simulink model "edma_single_block_transfer_profiling_s32k14x"  (Simulink 9.0)
settings: Solver=FixedStepDiscrete  StartTime=0.0  StopTime=10.0  FixedStep=2  RelTol=1e-3  EnableMultiTasking=on
model workspace (MAT data in the model file):
  dest = 1234
  sig_src = Simulink.Signal
  sig_src.DataType = 'uint32'
  sig_src.Dimensions = 1025
  sig_src.DimensionsMode = 'auto'
  sig_src.Complexity = 'auto'
  sig_src.SampleTime = -1
  sig_src.SamplingMode = 'auto'
InitFcn:
  | mbd_s32k_consistency_checks(bdroot(gcs));
undefined symbols (not defined in the file): LQFP
libraries: mbd_s32k1xx_ec_toolbox x8, simulink x1
Description:
  | Comparison betwen data transfer using eDMA and normal cpu copy.
  | 
  | Transfer sizes used are as follows:
  | 4, 8, 16, 32, 64, 128, 256, 512, 768, 1024 uint32s (multiply by 4 to get number of bytes)
  | 
  | Transfer size is changed at every step, iterating circulary over this list.
  | 
  | Verification:
  | Open freeMaster project (has the same name as the model) and observe differences betwen the 2 types of transfer.
settings Model: Creator=NXP MBDT Team  LastModifiedBy=nxf35172
settings DataIOCC: ExternalInput=off  InitialState=off  LimitDataPoints=on  SaveFormat=Dataset  SaveOutput=off  SignalLogging=off  SaveTime=off
settings OptimizationCC: DefaultParameterBehavior=Inlined  PassReuseOutputArgsAs=Individual arguments  LifeSpan=auto
settings DebuggingCC: UnderspecifiedInitializationDetection=Simplified  MergeDetectMultiDrivingBlocksExec=error  InheritedTsInSrcMsg=none  SingleTaskRateTransMsg=error  ParameterTunabilityLossMsg=error  UnconnectedInputMsg=error  UnconnectedOutputMsg=error  UnconnectedLineMsg=error  AllowSymbolicDim=off  UnknownTsInhSupMsg=error
settings HardwareCC: ProdLargestAtomicInteger=Long  ProdLargestAtomicFloat=Double  ProdIntDivRoundTo=Zero  ProdEndianess=LittleEndian  ProdHWDeviceType=ARM Compatible->ARM Cortex
settings SFSimCC: MATLABDynamicMemAlloc=off
settings RTWCC: SystemTargetFile=mbd_s32k.tlc  MakeCommand=mbd_s32k_make_rtw COPY_MDLREF_INCLUDES=0  TemplateMakefile=mbd_s32k.tmf  Description=Model Based Design Toolbox S32K14x Code Generation Target  GenerateReport=on  IncludeHyperlinkInReport=on  LaunchReport=on  GenerateTraceInfo=on  GenerateTraceReport=on  GenerateTraceReportSl=on  GenerateTraceReportSf=on  GenerateTraceReportEml=on
settings CodeAppCC: ForceParamTrailComments=on  IgnoreCustomStorageClasses=off  OperatorAnnotations=on  SimulinkDataObjDesc=on  SFDataObjDesc=on  InsertBlockDesc=on  StateflowObjectComments=off
settings STFCustomTargetCC: MultiwordLength=256  ModelReferenceCompliant=off  CombineOutputUpdateFcns=on  ERTCustomFileBanners=on  SupportContinuousTime=off  SupportNonInlinedSFcns=off  RemoveResetFunc=on  MATLABClassNameForMDSCustomization=Simulink.SoftwareTarget.ERTCustomization  GRTInterface=off  SystemTargetFile=mbd_s32k.tlc
settings ERTTargetCC: ModelReferenceCompliant=off  ParMdlRefBuildCompliant=off  CompOptLevelCompliant=off  ConcurrentExecutionCompliant=off  ModelStepFunctionPrototypeControlCompliant=off  CPPClassGenCompliant=off  UseToolchainInfoCompliant=off  InlinedParameterPlacement=NonHierarchical  ERTCustomFileTemplate=example_file_process.tlc

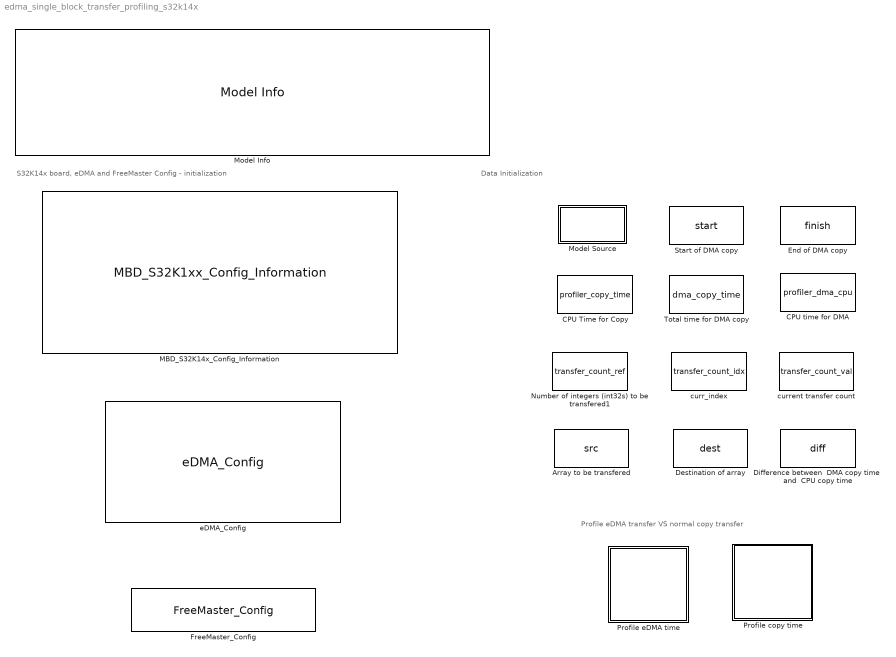
== system edma_single_block_transfer_profiling_s32k14x ==
  note: Profile eDMA transfer VS normal copy transfer
  note: S32K14x board, eDMA and FreeMaster Config - initialization
  note: Data Initialization
  Array to be transfered : DataStoreMemory  DataStoreName=src  ReadBeforeWriteMsg=warning  WriteAfterWriteMsg=warning  WriteAfterReadMsg=warning  ShowAdditionalParam=off
  CPU Time for Copy : DataStoreMemory  DataStoreName=profiler_copy_time  ReadBeforeWriteMsg=warning  WriteAfterWriteMsg=warning  WriteAfterReadMsg=warning  ShowAdditionalParam=off  OutDataTypeStr=uint32
  CPU time for DMA : DataStoreMemory  DataStoreName=profiler_dma_cpu  ReadBeforeWriteMsg=warning  WriteAfterWriteMsg=warning  WriteAfterReadMsg=warning  ShowAdditionalParam=off  OutDataTypeStr=uint32
  Destination of array : DataStoreMemory  DataStoreName=dest  ReadBeforeWriteMsg=warning  WriteAfterWriteMsg=warning  WriteAfterReadMsg=warning  ShowAdditionalParam=off
  Difference between  DMA copy time  and  CPU copy time : DataStoreMemory  DataStoreName=diff  ReadBeforeWriteMsg=warning  WriteAfterWriteMsg=warning  WriteAfterReadMsg=warning  ShowAdditionalParam=off  OutDataTypeStr=int32
  End of DMA copy : DataStoreMemory  DataStoreName=finish  ReadBeforeWriteMsg=warning  WriteAfterWriteMsg=warning  WriteAfterReadMsg=warning  ShowAdditionalParam=off
  FreeMaster_Config : mbd_s32k1xx_ec_toolbox/Utility Blocks/FreeMaster_Config  interface=LPUART1  baudrate=115200  rxd=PTC6: [LPUART1_RX | Receive]  txd=PTC7: [LPUART1_TX | Transmit]  mode=Short Interrupt  isr_prio=5  show_adv_opts=on  use_scope=on  max_scope_vars=8  use_recorder=on  max_rec_vars=8  rec_buff_size=1024  rec_timebase=0 milliseconds  comm_buffer_size_auto=on  comm_buffer_size=255  comm_rqueue_size_default=on  comm_rqueue_size=32
  MBD_S32K14x_Config_Information : mbd_s32k1xx_ec_toolbox/MBD_S32K1xx_Config_Information  Priority=1  mbdt_ver=0  disp_str=|  config_params=[]  mcu_target_name=S32K144  mcu_target_package=100-LQFP  mcu_target_sram_size=64KB  mcu_system_clock_freq=80  mcu_xtal_freq=External 8  mcu_steptick_timer=LPIT Channel 0  mcu_steptick_prio=15  ds_import_enable=on  target_compiler=GCC  target_memory=FLASH  gcc_target_compile_opts=-mcpu=cortex-m4 -mthumb -mfloat-abi=hard -mfpu=fpv4-sp-d16 -O1 -g -gstrict-dwarf  gcc_target_assemble_opts=-mcpu=cortex-m4 -mthumb -mfloat-abi=hard -mfpu=fpv4-sp-d16 -g  gcc_target_link_opts=-mcpu=cortex-m4 -mthumb -mfloat-abi=hard -mfpu=fpv4-sp-d16  gcc_target_default_lcf=on  gcc_target_user_lcf=S32K144_64_flash.ld  ghs_target_compile_opts=-cpu=cortexm4f -thumb -DARM_MATH_CM4 -fpu=vfpv4_d16 -fsingle -Ogeneral -Wundef -Wimplicit-int -Wshadow -Wtrigraphs --no_commons --gnu_asm -gnu99 -gdwarf-2 -G  ghs_target_assemble_opts=-cpu=cortexm4f -fpu=vfpv4_d16  ghs_target_link_opts=-cpu=cortexm4f -thumb -fpu=vfpv4_d16  ghs_target_default_lcf=off  ghs_target_user_lcf=S32K144_64_flash.ld  iar_target_compile_opts=--cpu=Cortex-M4F --thumb --fpu=VFPv4_sp -Ol -e --debug --dlib_config normal  iar_target_assemble_opts=--cpu Cortex-M4F --thumb --fpu VFPv4_sp  iar_target_link_opts=--no_exceptions --vfe --inline  iar_target_default_lcf=off  iar_target_user_lcf=S32K144_64_flash.icf  pil_download_enable=off  rbl_download_enable=on  rbl_start_delay=5000000  rbl_download_interface=OpenSDA  rbl_restart_request=off  rbl_com_port=Custom  rbl_com_port_custom=COM1  pil_download_rate=57600  pil_opensda_drive=Custom  pil_opensda_drive_custom=D  pil_uart_instance=0  pil_uart_rx=PTA2: [LPUART0_RX | Receive]  pil_uart_tx=PTA3: [LPUART0_TX | Transmit]  FTM_PWM_PcrCheckEnDis=on  FTM_Input_Edge_Inputs_PcrCheckEnDis=on  FTM_Dual_Edge_Inputs_PcrCheckEnDis=on  FTM_Quadrature_Inputs_PcrCheckEnDis=on  FTM_Hall_Sensor_Inputs_PcrCheckEnDis=on  LPTMR_PcrCheckEnDis=on  PIT_PcrCheckEnDis=on  RTC_PcrCheckEnDis=on  FlexCAN_PcrCheckEnDis=on  LIN_PcrCheckEnDis=on  FlexIO_PcrCheckEnDis=on  LPI2C_PcrCheckEnDis=on  LPSPI_PcrCheckEnDis=on  LPUART_PcrCheckEnDis=on  CMP_PcrCheckEnDis=on  GPIO_OutputPcrCheckEnDis=on  GPIO_InputPcrCheckEnDis=on  SBC_PcrCheckEnDis=on  AMMCLIB_PcrCheckEnDis=on  FM_PcrCheckEnDis=on  Profile_PcrCheckEnDis=on  ConfigParams_PcrCheckEnDis=on  ModelRef_PcrCheckEnDis=on  PDB0_PcrCheckEnDis=on  CSEc_PcrCheckEnDis=on  eDMA_PcrCheckEnDis=on  ADC_PcrCheckEnDis=on  WDOG_PcrCheckEnDis=on
      | Target : S32K144-64KB_SRAM
      | Package : 100-pin
      | System clock : 80 MHz
      | XTAL clock : External 8 MHz
      | Compiler : GCC
      | Target Type : FLASH
      | Download Code after build : off
      | Step Tick Interrupt Priority : 15
  Model Info : simulink/Model-Wide Utilities/Model Info  Frame=off  DisplayStringWithTags=|  HorizontalTextAlignment=Left  LeftAlignmentValue=0.02
      | Model Name: %<ModelName>
      | 
      | Description: %<Description>
  Model Source : Subsystem  mask(Model Source){ShowInLibBrowser=0}
      mask prompts: ShowInLibBrowser "Simulink:masks:CustCodeMaskParam1_MP"
      settings: CopyFcn=cccopyfcn(gcb)  OpenFcn=ccopenfcn('Model Source')
      mask Help: eval('feval(''rtwprivate'',''rtwhelpview'',''rtw_model_source_block'')');
      mask Display: disp('Model\nSource');
  Number of integers (int32s) to be transfered1 : DataStoreMemory  DataStoreName=transfer_count_ref  ReadBeforeWriteMsg=warning  WriteAfterWriteMsg=warning  WriteAfterReadMsg=warning  InitialValue=[4,8,16,32,64,128,256,512,768,1024]  ShowAdditionalParam=off  OutDataTypeStr=uint32
  Profile copy time : Subsystem  Priority=2
  Profile eDMA time : Subsystem  Priority=3
      settings: RTWSystemCode=Nonreusable function  FunctionWithSeparateData=on
  Start of DMA copy : DataStoreMemory  DataStoreName=start  ReadBeforeWriteMsg=warning  WriteAfterWriteMsg=warning  WriteAfterReadMsg=warning  ShowAdditionalParam=off
  Total time for DMA copy : DataStoreMemory  DataStoreName=dma_copy_time  ReadBeforeWriteMsg=warning  WriteAfterWriteMsg=warning  WriteAfterReadMsg=warning  ShowAdditionalParam=off
  curr_index : DataStoreMemory  DataStoreName=transfer_count_idx  ReadBeforeWriteMsg=warning  WriteAfterWriteMsg=warning  WriteAfterReadMsg=warning  ShowAdditionalParam=off  OutDataTypeStr=uint32
  current transfer count : DataStoreMemory  DataStoreName=transfer_count_val  ReadBeforeWriteMsg=warning  WriteAfterWriteMsg=warning  WriteAfterReadMsg=warning  ShowAdditionalParam=off  OutDataTypeStr=uint32
  eDMA_Config : mbd_s32k1xx_ec_toolbox/Core and System Blocks/DMA Blocks/eDMA_Config  Priority=2  channel=0  show_advanced_tab=on  channel_advanced_checkbox=on  show_enabled=on  arbitration=EDMA_ARBITRATION_FIXED_PRIORITY  halt_on_error=false  channel0priority=EDMA_CHN_DEFAULT_PRIORITY  channel0requestsource=EDMA_REQ_DISABLED  channel0enable=on  channel1priority=EDMA_CHN_DEFAULT_PRIORITY  channel1requestsource=EDMA_REQ_DISABLED  channel1enable=on  channel2priority=EDMA_CHN_DEFAULT_PRIORITY  channel2requestsource=EDMA_REQ_DISABLED  channel2enable=off  channel3priority=EDMA_CHN_DEFAULT_PRIORITY  channel3requestsource=EDMA_REQ_DISABLED  channel3enable=off  channel4priority=EDMA_CHN_DEFAULT_PRIORITY  channel4requestsource=EDMA_REQ_DISABLED  channel4enable=off  channel5priority=EDMA_CHN_DEFAULT_PRIORITY  channel5requestsource=EDMA_REQ_DISABLED  channel5enable=off  channel6priority=EDMA_CHN_DEFAULT_PRIORITY  channel6requestsource=EDMA_REQ_DISABLED  channel6enable=off  channel7priority=EDMA_CHN_DEFAULT_PRIORITY  channel7requestsource=EDMA_REQ_DISABLED  channel7enable=off  channel8priority=EDMA_CHN_DEFAULT_PRIORITY  channel8requestsource=EDMA_REQ_DISABLED  channel8enable=off  channel9priority=EDMA_CHN_DEFAULT_PRIORITY  channel9requestsource=EDMA_REQ_DISABLED  channel9enable=off  channel10priority=EDMA_CHN_DEFAULT_PRIORITY  channel10requestsource=EDMA_REQ_DISABLED  channel10enable=off  channel11priority=EDMA_CHN_DEFAULT_PRIORITY  channel11requestsource=EDMA_REQ_DISABLED  channel11enable=off  channel12priority=EDMA_CHN_DEFAULT_PRIORITY  channel12requestsource=EDMA_REQ_DISABLED  channel12enable=off  channel13priority=EDMA_CHN_DEFAULT_PRIORITY  channel13requestsource=EDMA_REQ_DISABLED  channel13enable=off  channel14priority=EDMA_CHN_DEFAULT_PRIORITY  channel14requestsource=EDMA_REQ_DISABLED  channel14enable=off  channel15priority=EDMA_CHN_DEFAULT_PRIORITY  channel15requestsource=EDMA_REQ_DISABLED  channel15enable=off

== system edma_single_block_transfer_profiling_s32k14x/Model Source ==

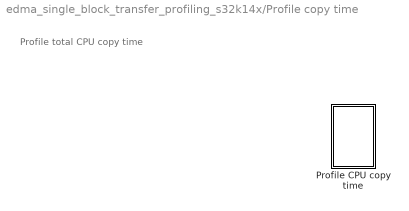
== system edma_single_block_transfer_profiling_s32k14x/Profile copy time ==
  note: Profile total CPU copy time
  Profile CPU copy time : Subsystem  TreatAsAtomicUnit=on

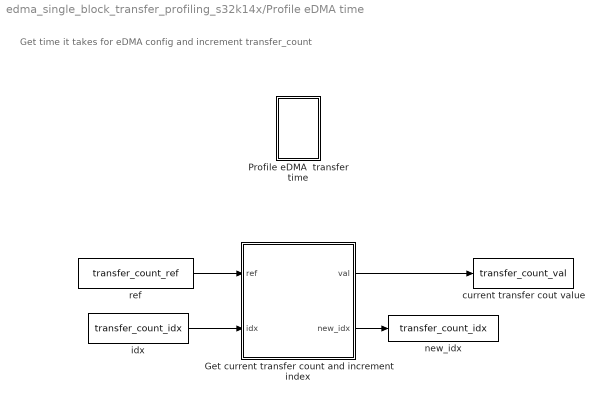
== system edma_single_block_transfer_profiling_s32k14x/Profile eDMA time ==
  note: Get time it takes for eDMA config and increment transfer_count
  Get current transfer count and increment index : MATLAB Function  TreatAsAtomicUnit=on
  Profile eDMA  transfer time : Subsystem  TreatAsAtomicUnit=on
      settings: RTWSystemCode=Nonreusable function  FunctionWithSeparateData=on
  current transfer cout value : DataStoreWrite  DataStoreName=transfer_count_val
  idx : DataStoreRead  DataStoreName=transfer_count_idx
  new_idx : DataStoreWrite  DataStoreName=transfer_count_idx
  ref : DataStoreRead  DataStoreName=transfer_count_ref
  wires:
  idx/1 -> Get current transfer count and increment index/2(idx)
  Get current transfer count and increment index/1(val) -> current transfer cout value/1
  Get current transfer count and increment index/2(new_idx) -> new_idx/1
  ref/1 -> Get current transfer count and increment index/1(ref)

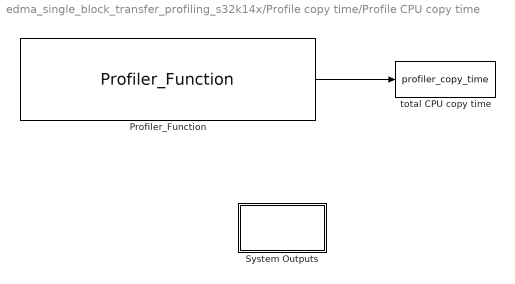
== system edma_single_block_transfer_profiling_s32k14x/Profile copy time/Profile CPU copy time ==
  Profiler_Function : mbd_s32k1xx_ec_toolbox/Utility Blocks/Profiler_Function  Priority=1  profile_indx=2
      settings: showOut=on
  System Outputs : Subsystem  Priority=12  mask(System Outputs){ShowInLibBrowser=0}
      mask prompts: ShowInLibBrowser "Simulink:masks:CustCodeMaskParam1_MP"
      settings: CopyFcn=cccopyfcn(gcb)  OpenFcn=ccopenfcn('System Outputs Function')  FunctionInterfaceSpec=Allow arguments  FunctionWithSeparateData=on
      mask Help: eval('feval(''rtwprivate'',''rtwhelpview'',''rtw_sys_outputs_block'')');
      mask Display: disp('System\nOutputs');
  total CPU copy time : DataStoreWrite  Priority=15  DataStoreName=profiler_copy_time
  wires:
  Profiler_Function/1 -> total CPU copy time/1

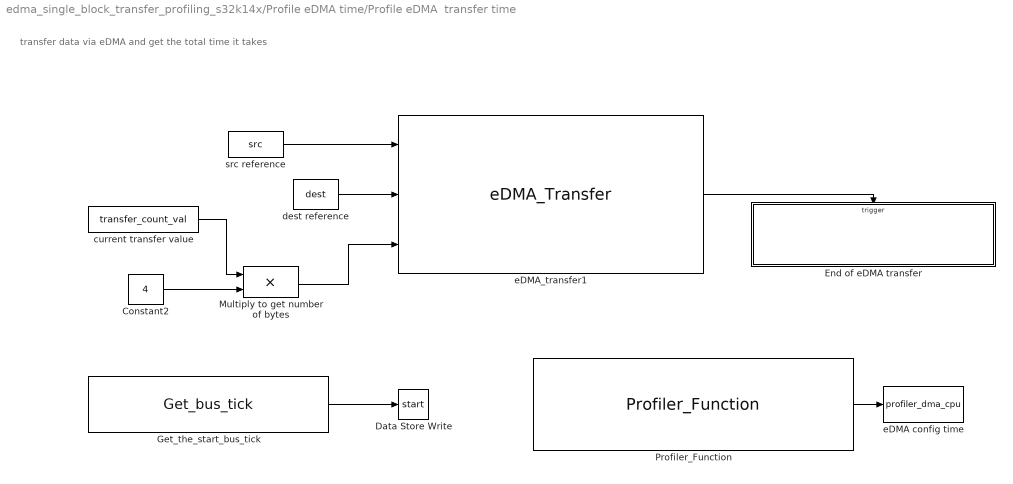
== system edma_single_block_transfer_profiling_s32k14x/Profile eDMA time/Profile eDMA  transfer time ==
  note: transfer data via eDMA and get the total time it takes
  Constant2 : Constant  Value=4  OutDataTypeStr=uint32
  Data Store Write : DataStoreWrite  DataStoreName=start
  End of eDMA transfer : Subsystem
  Get_the_start_bus_tick : mbd_s32k1xx_ec_toolbox/Utility Blocks/Get_bus_tick  Priority=1
  Multiply to get number of bytes : Product  Priority=2  OutDataTypeStr=uint32
  Profiler_Function : mbd_s32k1xx_ec_toolbox/Utility Blocks/Profiler_Function  profile_indx=0
      settings: showOut=on
  current transfer value : DataStoreRead  DataStoreName=transfer_count_val
  dest reference : DataStoreRead  Priority=2  DataStoreName=dest
  eDMA config time : DataStoreWrite  DataStoreName=profiler_dma_cpu
  eDMA_transfer1 : mbd_s32k1xx_ec_toolbox/Core and System Blocks/DMA Blocks/eDMA_Transfer  Priority=5  channel=0  transfer_mode=Single Block Transfer  transfer_type=EDMA_TRANSFER_MEM2MEM  transfer_size=EDMA_TRANSFER_SIZE_4B  single_block_src_type=Src input is an address  single_block_dest_type=Dest input is an address  bytes_on_each_req=4  sg_struct_size=32  src_list={32768, 1}  src_list_type=Value list  dest_list={PTD_BASE + 0xc, 0x400FF0CC}  dest_list_type=Address list  src_periph1=ADC0  src_reg1=SC1A  src_reg1offset=0  src_reg1enable=off  src_reg1_addr=0x4003B000  src_periph2=ADC0  src_reg2=SC1A  src_reg2offset=0  src_reg2enable=off  src_reg2_addr=0x4003B000  src_periph3=ADC0  src_reg3=SC1A  src_reg3offset=0  src_reg3enable=off  src_reg3_addr=0x4003B000  src_periph4=ADC0  src_reg4=SC1A  src_reg4offset=0  src_reg4enable=off  src_reg4_addr=0x4003B000  src_periph5=ADC0  src_reg5=SC1A  src_reg5offset=0  src_reg5enable=off  src_reg5_addr=0x4003B000  src_periph6=ADC0  src_reg6=SC1A  src_reg6offset=0  src_reg6enable=off  src_reg6_addr=0x4003B000  src_periph7=ADC0  src_reg7=SC1A  src_reg7offset=0  src_reg7enable=off  src_reg7_addr=0x4003B000  src_periph8=ADC0  src_reg8=SC1A  src_reg8offset=0  src_reg8enable=off  src_reg8_addr=0x4003B000  dest_periph1=ADC0  dest_reg1=SC1A  dest_reg1offset=0  dest_reg1enable=off  dest_reg1_addr=0x4003B000  dest_periph2=ADC0  dest_reg2=SC1A  dest_reg2offset=0  dest_reg2enable=off  dest_reg2_addr=0x4003B000  dest_periph3=ADC0  dest_reg3=SC1A  dest_reg3offset=0  dest_reg3enable=off  dest_reg3_addr=0x4003B000  dest_periph4=ADC0  dest_reg4=SC1A  dest_reg4offset=0  dest_reg4enable=off  dest_reg4_addr=0x4003B000  dest_periph5=ADC0  dest_reg5=SC1A  dest_reg5offset=0  dest_reg5enable=off  dest_reg5_addr=0x4003B000  dest_periph6=ADC0  dest_reg6=SC1A  dest_reg6offset=0  dest_reg6enable=off  dest_reg6_addr=0x4003B000  dest_periph7=ADC0  dest_reg7=SC1A  dest_reg7offset=0  dest_reg7enable=off  dest_reg7_addr=0x4003B000  dest_periph8=ADC0  dest_reg8=SC1A  dest_reg8offset=0  dest_reg8enable=off  dest_reg8_addr=0x4003B000
  src reference : DataStoreRead  Priority=2  DataStoreName=src
  wires:
  dest reference/1 -> eDMA_transfer1/2
  src reference/1 -> eDMA_transfer1/1
  current transfer value/1 -> Multiply to get number of bytes/1
  Constant2/1 -> Multiply to get number of bytes/2
  Multiply to get number of bytes/1 -> eDMA_transfer1/3
  eDMA_transfer1/1 -> End of eDMA transfer/Trigger
  Get_the_start_bus_tick/1 -> Data Store Write/1
  Profiler_Function/1 -> eDMA config time/1

== system edma_single_block_transfer_profiling_s32k14x/Profile copy time/Profile CPU copy time/System Outputs ==

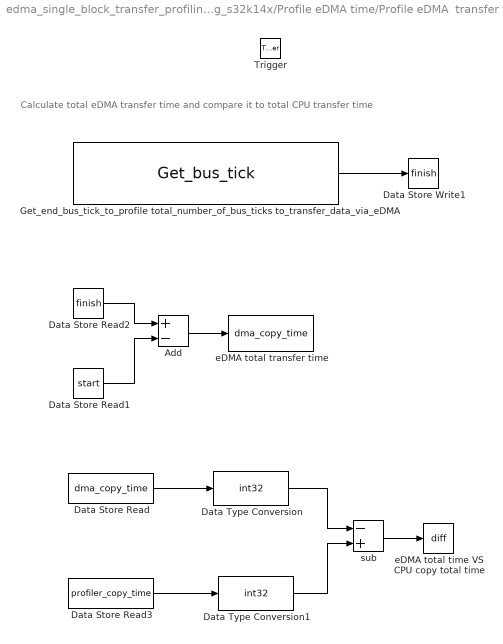
== system edma_single_block_transfer_profiling_s32k14x/Profile eDMA time/Profile eDMA  transfer time/End of eDMA transfer ==
  note: Calculate total eDMA transfer time and compare it to total CPU transfer time
  Trigger : TriggerPort  TriggerType=function-call  VariantControl=Variant  PortDimensions=1
  Add : Sum  Priority=5  Inputs=+-
  Data Store Read : DataStoreRead  DataStoreName=dma_copy_time
  Data Store Read1 : DataStoreRead  DataStoreName=start
  Data Store Read2 : DataStoreRead  DataStoreName=finish
  Data Store Read3 : DataStoreRead  DataStoreName=profiler_copy_time
  Data Store Write1 : DataStoreWrite  DataStoreName=finish
  Data Type Conversion : DataTypeConversion  OutDataTypeStr=int32
  Data Type Conversion1 : DataTypeConversion  OutDataTypeStr=int32
  Get_end_bus_tick_to_profile total_number_of_bus_ticks to_transfer_data_via_eDMA : mbd_s32k1xx_ec_toolbox/Utility Blocks/Get_bus_tick  Priority=1
  eDMA total transfer time : DataStoreWrite  DataStoreName=dma_copy_time
  eDMA total time VS CPU copy total time : DataStoreWrite  DataStoreName=diff
  sub : Sum  Priority=5  Inputs=-+
  wires:
  Get_end_bus_tick_to_profile total_number_of_bus_ticks to_transfer_data_via_eDMA/1 -> Data Store Write1/1
  Data Store Read2/1 -> Add/1
  Data Store Read1/1 -> Add/2
  Add/1 -> eDMA total transfer time/1
  sub/1 -> eDMA total time VS CPU copy total time/1
  Data Store Read/1 -> Data Type Conversion/1
  Data Type Conversion/1 -> sub/1
  Data Store Read3/1 -> Data Type Conversion1/1
  Data Type Conversion1/1 -> sub/2

== matlab function Profile eDMA time/Get current transfer count and increment index ==
  data: ref input double; val output double; idx input double; new_idx output double
function [val, new_idx] = fcn(ref, idx)
%#codegen
    new_idx = mod(idx, 10) + 1;
    val = ref(new_idx);
end
